simulink model "DC_Motor_v1"  (R2018b)
settings: Solver=VariableStepAuto  StartTime=0.0  StopTime=10.0  RelTol=1e-3
values from neighbouring files (symbols this model uses):
  b = 22.5    [DC_Simulink.m]
  K = 0.055    [DC_Servomotor_Code.m]    (also in DC_Simulink.m = 0.109)
  L = 5.02E-3    (= 0.00502)    [DC_Servomotor_Code.m]    (also in DC_Simulink.m = 0.000625)
  R = 41.5    [DC_Servomotor_Code.m]    (also in DC_Simulink.m = 0.522)
undefined symbols (not defined in the file or in its folder): Gain, j
settings Model: Creator=james.quan.166  LastModifiedBy=james.quan.166

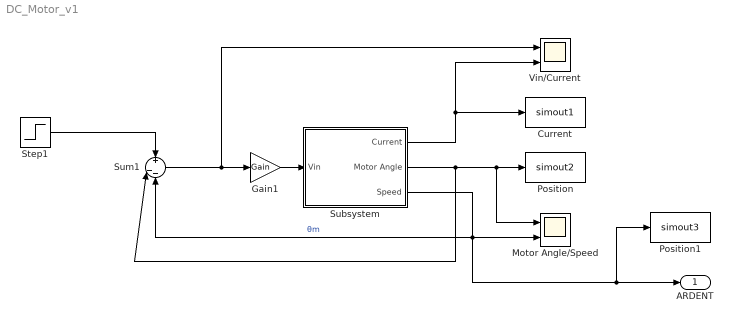
== system DC_Motor_v1 ==
  Current : ToWorkspace  VariableName=simout1  SaveFormat=Timeseries  SampleTime=-1
  Gain1 : Gain  Gain=Gain
  Motor Angle/Speed : Scope  NumInputPorts=2
  Position : ToWorkspace  VariableName=simout2  SaveFormat=Timeseries  SampleTime=-1
  Position1 : ToWorkspace  VariableName=simout3  SaveFormat=Timeseries  SampleTime=-1
  Step1 : Step  After=10  SampleTime=0
  Subsystem : Subsystem
  Sum1 : Sum  Inputs=+|--
  Vin/Current : Scope  NumInputPorts=2
  ARDENT : Outport
  wires:
  Subsystem/2(Motor Angle) -> Motor Angle/Speed/1, Position/1, Sum1/2
  Step1/1 -> Sum1/1
  Gain1/1 -> Subsystem/1(Vin)
  Subsystem/1(Current) -> Vin/Current/2, Current/1
  Subsystem/3(Speed) -> Sum1/3, Position1/1, ARDENT/1, Motor Angle/Speed/2  "θm"
  Sum1/1 -> Vin/Current/1, Gain1/1

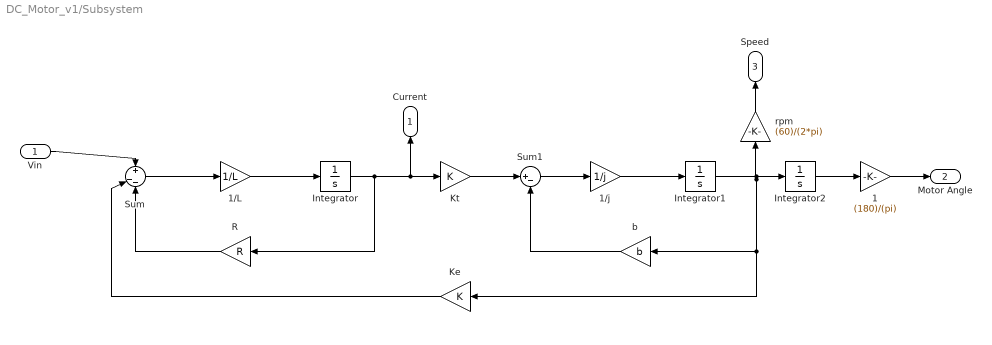
== system DC_Motor_v1/Subsystem ==
  Vin : Inport
  1 : Gain  Gain=(180)/(pi)
  1/L : Gain  Gain=1/L
  1/j : Gain  Gain=1/j
  Integrator : Integrator
  Integrator1 : Integrator
  Integrator2 : Integrator
  Ke : Gain  Gain=K
  "Kt " : Gain  Gain=K
  R : Gain  Gain=R
  Sum : Sum  Inputs=+|--
  Sum1 : Sum  Inputs=|+-
  "b " : Gain  Gain=b
  rpm : Gain  Gain=(60)/(2*pi)
  Current : Outport
  Motor Angle : Outport  Port=2
  Speed : Outport  Port=3
  wires:
  Integrator2/1 -> 1/1
  1/j/1 -> Integrator1/1
  "b "/1 -> Sum1/2
  1/L/1 -> Integrator/1
  Sum1/1 -> 1/j/1
  "Kt "/1 -> Sum1/1
  Sum/1 -> 1/L/1
  Integrator1/1 -> Integrator2/1, rpm/1, Ke/1, "b "/1
  Vin/1 -> Sum/1
  Ke/1 -> Sum/2
  R/1 -> Sum/3
  Integrator/1 -> Current/1, "Kt "/1, R/1
  rpm/1 -> Speed/1
  1/1 -> Motor Angle/1
